simulink model "mbd3_01"  (R2020b)
settings: Solver=VariableStepAuto  StartTime=0.0  StopTime=10.0  RelTol=1e-3
settings Model: Creator=karth  LastModifiedBy=karth

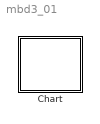
== system mbd3_01 ==
  Chart : Stateflow chart  TreatAsAtomicUnit=on

== stateflow chart mbd3_01/Chart ==
  state Stop
    y1=Red;
    y2=Green;
  state SopForTraffic
    y1=Red;
    y2=Green;
  state StopToGo
    y1=Red;
    y2=Green;
  note: after(20,tick)
  note: [sens]
  note: after(3,tick)
  state GoToStop
    y1=Yellow;
    y2=Red;
  state Go
    y1=Green;
    y2=Red;
  note: after(10,tick)
  (default) -> Stop
  Stop -> SopForTraffic
  SopForTraffic -> StopToGo
  GoToStop -> Stop
  StopToGo -> Go
  Go -> GoToStop
